simulink model "Generic_Aero_Piston_Digital_Twin"  (R2026a)
settings: Solver=VariableStepAuto  StopTime=30
libraries: SignalEditorBlockLib x3
settings Model: Creator=bhanu  LastModifiedBy=bhanu

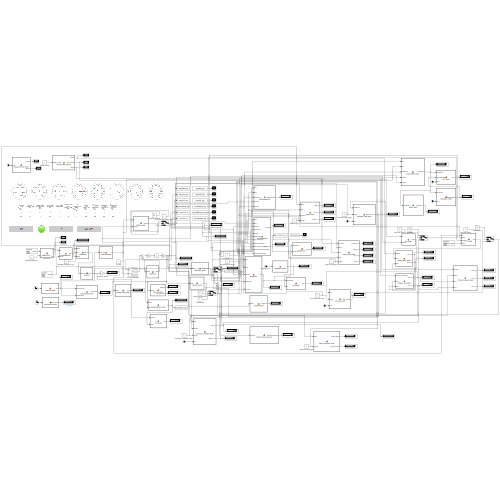
[thumbnail: Simulink's stored preview of the top-level diagram]
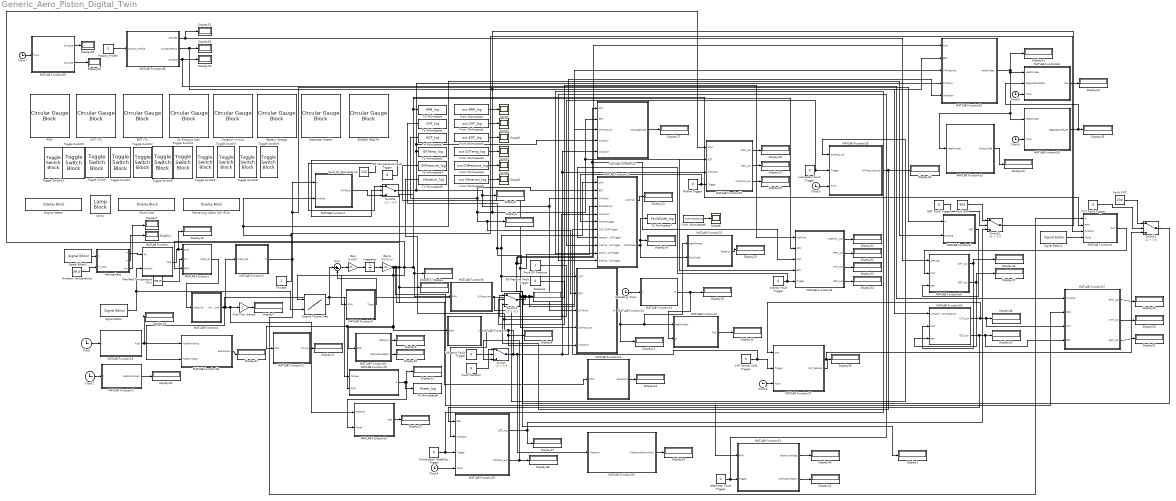
== system Generic_Aero_Piston_Digital_Twin ==
  " Fault Code" : DisplayBlock  LabelPosition=Hide  Transparency=1  GridColor=[0.502, 0.502, 0.502]
  Alternator Fault Trigger : Constant  Value=0
  Alternator Health : CircularGaugeBlock  LabelPosition=Hide  FontColor=[0.0, 0.0, 0.0]
  Ambient Temperature : Constant  Value=288.15
  Atmosphere : MATLAB Function  TreatAsAtomicUnit=on
  Battery Voltage : CircularGaugeBlock  LabelPosition=Hide  ScaleMax=16  FontColor=[0.0, 0.0, 0.0]
  CHT (°C) : CircularGaugeBlock  Description=CHT  LabelPosition=Hide  ScaleMax=150  FontColor=[0.0, 0.0, 0.0]
  CHT Fault Trigger : Constant  Value=0
  CHT Sensor Drift Trigger : Constant  Value=0
  Clock{,1..7} (8 alike) : Clock
  Combustion Instability Trigger : Constant  Value=0
  Display{,1..56} (57 alike) : Display
  EGT (°C) : CircularGaugeBlock  LabelPosition=Hide  ScaleMax=1000  FontColor=[0.0, 0.0, 0.0]
  EGT Fault Trigger : Constant  Value=0
  ENGINE HEALTH : CircularGaugeBlock  LabelPosition=Hide  FontColor=[0.0, 0.0, 0.0]
  "Engine Health  " : DisplayBlock  LabelPosition=Hide  Transparency=1  GridColor=[0.502, 0.502, 0.502]
  Engine Torque Map : Lookup_n-D  BreakpointsForDimension1=[3500 4000 4500 5000 5500 5800]  BreakpointsForDimension2=[0 0.25 0.5 0.75 1]  Table=|  InternalRulePriority=Speed  RndMeth=Simplest
      | [20 35 55 80 100;
      |  20 40 60 85 110;
      |  18 42 65 90 118;
      |  18 45 70 100 125;
      |  18 45 72 102 127.6;
      |  15 42 68 98 120]
      settings: InputPortMap=u0,u1
  Fault CHT : Constant  Value=130
  Fault EGT : Constant  Value=900
  Fault Oil Pressure : Constant
  Fault Oil Temperature : Constant  Value=120
  Fault Vibration : Constant  Value=5
  From Workspace : FromWorkspace  VariableName=out.RPM_log
  From Workspace1 : FromWorkspace  VariableName=out.CHT_log
  From Workspace2 : FromWorkspace  VariableName=out.EGT_log
  From Workspace3 : FromWorkspace  VariableName=out.OilTemp_log
  From Workspace4 : FromWorkspace  VariableName=out.OilPressure_log
  From Workspace5 : FromWorkspace  VariableName=out.Vibration_log
  From Workspace6 : FromWorkspace  VariableName=out.FaultCode_log
  Fuel Flow Sensor : Gain
  Gain : Gain  Gain=6.6667
  Gain1 : Gain  Gain=60/(2*pi)
  Injector Fault Trigger : Constant  Value=0
  Integrator : Integrator  InitialCondition=575.96
  Lamp : LampBlock  LabelPosition=Hide  DefaultColor=[192.0, 192.0, 192.0]
  Lubrication Fault Trigger : Constant  Value=0
  MATLAB Function : MATLAB Function  TreatAsAtomicUnit=on
  MATLAB Function1 : MATLAB Function  TreatAsAtomicUnit=on
  MATLAB Function10 : MATLAB Function  TreatAsAtomicUnit=on
  MATLAB Function11 : MATLAB Function  TreatAsAtomicUnit=on
  MATLAB Function12 : MATLAB Function  TreatAsAtomicUnit=on
  MATLAB Function13 : MATLAB Function  TreatAsAtomicUnit=on
  MATLAB Function14 : MATLAB Function  TreatAsAtomicUnit=on
  MATLAB Function15 : MATLAB Function  TreatAsAtomicUnit=on
  MATLAB Function16 : MATLAB Function  TreatAsAtomicUnit=on
  MATLAB Function17 : MATLAB Function  TreatAsAtomicUnit=on
  MATLAB Function18 : MATLAB Function  TreatAsAtomicUnit=on
  MATLAB Function19 : MATLAB Function  TreatAsAtomicUnit=on
  MATLAB Function2 : MATLAB Function  TreatAsAtomicUnit=on
  MATLAB Function20 : MATLAB Function  TreatAsAtomicUnit=on
  MATLAB Function21 : MATLAB Function  TreatAsAtomicUnit=on
  MATLAB Function22 : MATLAB Function  TreatAsAtomicUnit=on
  MATLAB Function23 : MATLAB Function  TreatAsAtomicUnit=on
  MATLAB Function24 : MATLAB Function  TreatAsAtomicUnit=on
  MATLAB Function25 : MATLAB Function  TreatAsAtomicUnit=on
  MATLAB Function26 : MATLAB Function  TreatAsAtomicUnit=on
  MATLAB Function27 : MATLAB Function  TreatAsAtomicUnit=on
  MATLAB Function28 : MATLAB Function  TreatAsAtomicUnit=on
  MATLAB Function29 : MATLAB Function  TreatAsAtomicUnit=on
  MATLAB Function3 : MATLAB Function  TreatAsAtomicUnit=on
  MATLAB Function30 : MATLAB Function  TreatAsAtomicUnit=on
  MATLAB Function31 : MATLAB Function  TreatAsAtomicUnit=on
  MATLAB Function32 : MATLAB Function  TreatAsAtomicUnit=on
  MATLAB Function33 : MATLAB Function  TreatAsAtomicUnit=on
  MATLAB Function34 : MATLAB Function  TreatAsAtomicUnit=on
  MATLAB Function35 : MATLAB Function  TreatAsAtomicUnit=on
  MATLAB Function36 : MATLAB Function  TreatAsAtomicUnit=on
  MATLAB Function37 : MATLAB Function  TreatAsAtomicUnit=on
  MATLAB Function38 : MATLAB Function  TreatAsAtomicUnit=on
  MATLAB Function39 : MATLAB Function  TreatAsAtomicUnit=on
  MATLAB Function4 : MATLAB Function  TreatAsAtomicUnit=on
  MATLAB Function5 : MATLAB Function  TreatAsAtomicUnit=on
  MATLAB Function6 : MATLAB Function  TreatAsAtomicUnit=on
  MATLAB Function7 : MATLAB Function  TreatAsAtomicUnit=on
  MATLAB Function8 : MATLAB Function  TreatAsAtomicUnit=on
  MATLAB Function9 : MATLAB Function  TreatAsAtomicUnit=on
  Manifold Temperature (Tm) : Constant  Value=288.15
  Misfire Trigger : Constant  Value=0
  Mission_Profile : Constant  Value=2
  Oil Pressure (bar) : CircularGaugeBlock  LabelPosition=Hide  ScaleMax=6  FontColor=[0.0, 0.0, 0.0]
  Oil Pressure Fault Trigger : Constant  Value=0
  Oil Temperature Fault Trigger : Constant  Value=0
  Operating Time : Clock
  RPM : CircularGaugeBlock  Tag=RPM  LabelPosition=Hide  ScaleMax=6000  FontColor=[0.0, 0.0, 0.0]
  Remaining Useful Life (RUL) : DisplayBlock  LabelPosition=Hide  Transparency=1  GridColor=[0.502, 0.502, 0.502]
  Scope{,1..6} (7 alike) : Scope
      Scope settings: ActiveDisplayYMinimum=3492.7664069639277  ActiveDisplayYMaximum=5723.0402452178787
      Scope1 settings: ActiveDisplayYMinimum=46.717948241029276  ActiveDisplayYMaximum=72.103645266326225
      Scope2 settings: ActiveDisplayYMinimum=420.76922361543927  ActiveDisplayYMaximum=801.55467899489327  DataLoggingVariableName=ScopeData2
      Scope3 settings: ActiveDisplayYMinimum=10  ActiveDisplayYMaximum=210  DataLoggingVariableName=ScopeData3
      Scope4 settings: ActiveDisplayYMinimum=3.4945760109784914  ActiveDisplayYMaximum=5.1672693321135013  DataLoggingVariableName=ScopeData4
      Scope5 settings: ActiveDisplayYMinimum=1.6286979532535071  ActiveDisplayYMaximum=2.0301472441392181  DataLoggingVariableName=ScopeData5
      Scope6 settings: ActiveDisplayYMinimum=-0.2207253886010363  ActiveDisplayYMaximum=0.19585492227979273  DataLoggingVariableName=ScopeData6
  Signal Editor : SignalEditorBlockLib/Signal Editor  FileName=C:\Users\bhanu\Documents\MATLAB\digital twin.mat  ActiveScenario=Scenario  ActiveSignal=Throttle  IsBus=off  OutputBusObjectStr=Bus: BusObject  SampleTime=0  ZeroCross=off  OutputAfterFinalValue=Setting to zero  Unit=inherit  PreserveSignalName=on  ApplySigPropsToAllScenarios=on  ApplySigPropsToAllSignals=off  SignalPropertySource=Dialog parameters
  Signal Editor1 : SignalEditorBlockLib/Signal Editor  FileName=C:\Users\bhanu\Documents\MATLAB\Amb Temp.mat  ActiveScenario=Scenario  ActiveSignal=Ambient Temp  IsBus=off  OutputBusObjectStr=Bus: BusObject  SampleTime=0  ZeroCross=off  OutputAfterFinalValue=Setting to zero  Unit=inherit  PreserveSignalName=on  ApplySigPropsToAllScenarios=on  ApplySigPropsToAllSignals=off  SignalPropertySource=Dialog parameters
  Signal Editor2 : SignalEditorBlockLib/Signal Editor  FileName=C:\Users\bhanu\Documents\MATLAB\Altitude.mat  ActiveScenario=Scenario  ActiveSignal=Altitude  IsBus=off  OutputBusObjectStr=Bus: BusObject  SampleTime=0  ZeroCross=off  OutputAfterFinalValue=Setting to zero  Unit=inherit  PreserveSignalName=on  ApplySigPropsToAllScenarios=on  ApplySigPropsToAllSignals=off  SignalPropertySource=Dialog parameters
  Sum : Sum  Inputs=|+-
  Switch{,1..4} (5 alike) : Switch  Criteria=u2 > Threshold  Threshold=0.5  SaturateOnIntegerOverflow=off  InputSameDT=off
  Throttle : Constant
  To Workspace : ToWorkspace  VariableName=RPM_log  SaveFormat=Timeseries  SampleTime=-1
  To Workspace1 : ToWorkspace  VariableName=CHT_log  SaveFormat=Timeseries  SampleTime=-1
  To Workspace2 : ToWorkspace  VariableName=EGT_log  SaveFormat=Timeseries  SampleTime=-1
  To Workspace3 : ToWorkspace  VariableName=OilTemp_log  SaveFormat=Timeseries  SampleTime=-1
  To Workspace4 : ToWorkspace  VariableName=OilPressure_log  SaveFormat=Timeseries  SampleTime=-1
  To Workspace5 : ToWorkspace  VariableName=Vibration_log  SaveFormat=Timeseries  SampleTime=-1
  To Workspace6 : ToWorkspace  VariableName=Power_log  SaveFormat=Timeseries  SampleTime=-1
  To Workspace7 : ToWorkspace  VariableName=FaultCode_log  SaveFormat=Timeseries  SampleTime=-1
  Toggle Switch{,1..10} (11 alike) : ToggleSwitchBlock
  Vibration (mm/s) : CircularGaugeBlock  LabelPosition=Hide  ScaleMax=5  FontColor=[0.0, 0.0, 0.0]
  Vibration Fault Trigger : Constant  Value=0
  wires:
  Ambient Temperature/1 -> Atmosphere/2(T_input)
  Atmosphere/1(P) -> MATLAB Function/1(Pa)
  Atmosphere/2(T) -> Display1/1
  Atmosphere/3(rho) -> Display2/1
  MATLAB Function/1(MAP) -> Display18/1, MATLAB Function1/1(MAP)
  Manifold Temperature (Tm)/1 -> MATLAB Function1/2(Tm)
  MATLAB Function1/1(mdot_air) -> MATLAB Function2/1(mdot_air)
  MATLAB Function2/1(mdot_fuel) -> MATLAB Function26/1(FuelFlow), MATLAB Function18/2(FuelBurnRate), MATLAB Function20/1(FuelFlow), Fuel Flow Sensor/1, MATLAB Function3/1(mdot_fuel)
  Engine Torque Map/1 -> Sum/1, MATLAB Function19/1(Torque)
  Sum/1 -> Gain/1
  Gain/1 -> Integrator/1
  Integrator/1 -> Gain1/1
  Gain1/1 -> MATLAB Function9/1(RPM), MATLAB Function10/1(RPM), MATLAB Function19/2(RPM), MATLAB Function11/1(RPM), MATLAB Function5/1(RPM), MATLAB Function37/2(RPM), MATLAB Function31/1(RPM), MATLAB Function25/1(RPM), Display17/1, MATLAB Function21/1(RPM), Engine Torque Map/1, MATLAB Function1/3(RPM), MATLAB Function4/2(RPM), To Workspace/1, MATLAB Function8/1(RPM), Display/1, MATLAB Function26/2(RPM)
  MATLAB Function5/1(Tload) -> Sum/2
  Throttle/1 -> MATLAB Function7/2(throttle), MATLAB Function6/2(throttle), MATLAB Function4/3(throttle)
  MATLAB Function3/1(P) -> MATLAB Function7/1(P), MATLAB Function6/1(P), MATLAB Function4/1(P)
  Switch1/1 -> MATLAB Function32/1(CHT), MATLAB Function23/1(CHT), MATLAB Function26/3(CHT), To Workspace1/1, MATLAB Function12/1(CHT), Display3/1, MATLAB Function13/1(CHT)
  Switch2/1 -> MATLAB Function12/2(EGT), Display4/1, MATLAB Function13/2(EGT), To Workspace2/1, MATLAB Function23/2(EGT), MATLAB Function25/2(EGT), MATLAB Function26/4(EGT), MATLAB Function32/2(EGT)
  Switch4/1 -> MATLAB Function32/4(OilTemp), MATLAB Function23/4(OilTemp), To Workspace3/1, MATLAB Function12/3(OilTemp), MATLAB Function13/3(OilTemp), Display5/1
  Switch3/1 -> To Workspace4/1, MATLAB Function13/4(OilPressure), MATLAB Function12/4(OilPressure), MATLAB Function23/3(OilPressure), MATLAB Function32/3(OilPressure), Display6/1
  Fuel Flow Sensor/1 -> Display7/1
  Switch/1 -> MATLAB Function32/5(Vibration), MATLAB Function25/3(Vibration), MATLAB Function23/5(Vibration), MATLAB Function30/1(Vibration), To Workspace5/1, MATLAB Function13/5(Vibration), MATLAB Function12/5(Vibration), Display8/1
  MATLAB Function10/1(BatteryV) -> Display9/1
  MATLAB Function10/2(AlternatorHealth) -> Display10/1
  MATLAB Function11/1(timing) -> Display11/1
  MATLAB Function12/1(HI) -> MATLAB Function22/1(HealthIndex), MATLAB Function14/1(HealthIndex), Display12/1
  MATLAB Function13/1(Anomaly) -> Display13/1
  MATLAB Function13/2(FaultCode) -> To Workspace7/1, Display14/1, MATLAB Function22/2(FaultCode)
  MATLAB Function14/1(RUL) -> Display15/1
  Operating Time/1 -> MATLAB Function15/1(t)
  MATLAB Function15/1(D) -> MATLAB Function14/2(D), Display16/1
  Signal Editor/1 -> Engine Torque Map/2, MATLAB Function/2(throttle)
  From Workspace/1 -> Scope/1
  From Workspace1/1 -> Scope1/1
  From Workspace2/1 -> Scope2/1
  From Workspace3/1 -> Scope3/1
  From Workspace4/1 -> Scope4/1
  From Workspace5/1 -> Scope5/1
  Signal Editor1/1 -> MATLAB Function4/4(Tamb)
  Signal Editor2/1 -> Atmosphere/1(h)
  Clock/1 -> MATLAB Function16/1(t)
  MATLAB Function16/1(Fuel) -> Display19/1, MATLAB Function18/1(FuelRemaining)
  Clock1/1 -> MATLAB Function17/1(t)
  MATLAB Function17/1(FuelConsumed) -> Display20/1
  MATLAB Function18/1(Endurance) -> Display21/1
  MATLAB Function19/1(P) -> MATLAB Function20/2(Power), Display22/1, To Workspace6/1
  MATLAB Function20/1(SFC) -> Display23/1
  MATLAB Function21/1(Response) -> Display24/1
  MATLAB Function22/1(Severity) -> Display25/1
  From Workspace6/1 -> Scope6/1
  Vibration Fault Trigger/1 -> Switch/2
  Fault Vibration/1 -> Switch/1
  Fault CHT/1 -> Switch1/1
  CHT Fault Trigger/1 -> Switch1/2
  Fault EGT/1 -> Switch2/1
  EGT Fault Trigger/1 -> Switch2/2
  Fault Oil Pressure/1 -> Switch3/1
  Oil Pressure Fault Trigger/1 -> Switch3/2
  MATLAB Function7/1(OilTemp) -> Switch4/3
  Fault Oil Temperature/1 -> Switch4/1
  Oil Temperature Fault Trigger/1 -> Switch4/2
  MATLAB Function23/1(MessageCode) -> Display27/1
  Misfire Trigger/1 -> MATLAB Function13/6(MisfireTrigger), MATLAB Function25/4(Trigger)
  MATLAB Function25/1(RPM_out) -> Display28/1
  MATLAB Function25/3(Vibration_out) -> Display30/1
  MATLAB Function25/2(EGT_out) -> Display29/1
  Injector Fault Trigger/1 -> MATLAB Function13/8(InjectorFaultTrigger), MATLAB Function26/5(Trigger)
  MATLAB Function26/1(FuelFlow_out) -> Display31/1
  MATLAB Function26/4(EGT_out) -> Display34/1
  MATLAB Function26/3(CHT_out) -> Display33/1
  MATLAB Function26/2(RPM_out) -> Display32/1
  CHT Sensor Drift Trigger/1 -> MATLAB Function13/7(CHT_DriftTrigger), MATLAB Function27/2(Trigger)
  Clock2/1 -> MATLAB Function27/3(Time)
  MATLAB Function27/1(CHT_Sensed) -> Switch1/3, Display35/1
  Lubrication Fault Trigger/1 -> MATLAB Function13/9(LubricationFaultTrigger), MATLAB Function28/2(Trigger)
  Clock3/1 -> MATLAB Function28/3(Time)
  MATLAB Function8/1(OilPressure) -> MATLAB Function28/1(OilPressure)
  MATLAB Function28/1(OilPressure_out) -> Display36/1, Switch3/3
  Combustion Instability Trigger/1 -> MATLAB Function13/10(CombustionInstabilityTrigger), MATLAB Function29/3(Trigger)
  MATLAB Function29/1(EGT_out) -> Display37/1, Switch2/3
  Clock4/1 -> MATLAB Function29/4(Time)
  MATLAB Function9/1(V) -> MATLAB Function29/2(Vibration)
  MATLAB Function29/2(Vibration_out) -> Switch/3, Display38/1
  MATLAB Function30/1(VibrationPatternFault) -> Display39/1
  Alternator Fault Trigger/1 -> MATLAB Function13/11(AlternatorFaultTrigger), MATLAB Function31/2(Trigger)
  MATLAB Function31/2(AlternatorHealth) -> Display41/1
  MATLAB Function31/1(BatteryVoltage) -> Display40/1
  MATLAB Function32/1(HealthIndex) -> MATLAB Function35/1(HealthIndex), MATLAB Function33/1(HealthIndex), MATLAB Function34/1(HealthIndex), Display42/1
  MATLAB Function33/1(StatusCode) -> Display43/1
  MATLAB Function34/1(RUL) -> Display44/1
  Clock5/1 -> MATLAB Function35/2(Time)
  MATLAB Function35/1(DegradationRate) -> MATLAB Function34/2(DegradationRate), Display45/1
  Clock6/1 -> MATLAB Function34/3(Time)
  MATLAB Function36/1(CHT_out) -> MATLAB Function24/2(CHT), Display46/1
  MATLAB Function36/2(EGT_out) -> MATLAB Function24/3(EGT), Display47/1
  MATLAB Function4/1(CHT) -> MATLAB Function36/2(CHT)
  MATLAB Function6/1(EGT) -> MATLAB Function36/3(EGT)
  MATLAB Function24/1(CHT_out) -> MATLAB Function27/1(CHT), MATLAB Function37/3(CHT), Display48/1
  MATLAB Function24/2(EGT_out) -> MATLAB Function29/1(EGT), MATLAB Function37/4(EGT), Display26/1
  MATLAB Function37/1(RPM_out) -> Display49/1
  MATLAB Function37/2(CHT_out) -> Display50/1
  MATLAB Function37/3(EGT_out) -> Display51/1
  Mission_Profile/1 -> MATLAB Function38/1(Mission_Profile)
  MATLAB Function38/2(AmbientTemp) -> Display53/1, MATLAB Function24/1(Ambient_Temperature)
  MATLAB Function38/3(Throttle) -> MATLAB Function37/1(Throttle), Display54/1
  MATLAB Function38/1(Altitude) -> Display52/1, MATLAB Function36/1(Altitude)
  Clock7/1 -> MATLAB Function39/1(Time)
  MATLAB Function39/1(Throttle) -> Display55/1
  MATLAB Function39/2(Altitude) -> Display56/1

== matlab function Generic_Aero_Piston_Digital_Twin/MATLAB Function10 ==
  data: RPM input; BatteryV output; AlternatorHealth output
function [BatteryV, AlternatorHealth] = Electrical_Model(RPM)

BatteryV = 24;

if RPM >= 1500
    AlternatorHealth = 100;
else
    AlternatorHealth = 50;
end

== matlab function Generic_Aero_Piston_Digital_Twin/MATLAB Function11 ==
  data: RPM input; timing output
function timing = InjectionTiming_Model(RPM)

timing_base = 25;      % degrees BTDC
timing = timing_base + 0.001*(RPM - 5500);

== matlab function Generic_Aero_Piston_Digital_Twin/MATLAB Function12 ==
  data: CHT input; HI output; EGT input; OilTemp input; OilPressure input; Vibration input
function HI = HealthIndex(CHT, EGT, OilTemp, OilPressure, Vibration)

HI = 100;

if CHT > 120
    HI = HI - 15;
end

if EGT > 850
    HI = HI - 15;
end

if OilTemp > 110
    HI = HI - 10;
end

if OilPressure < 2
    HI = HI - 20;
end

if Vibration > 4
    HI = HI - 20;
end

HI = max(0,HI);

== matlab function Generic_Aero_Piston_Digital_Twin/MATLAB Function13 ==
  data: CHT input; Anomaly output; EGT input; OilTemp input; OilPressure input; Vibration input; FaultCode output; MisfireTrigger input; CHT_DriftTrigger input; InjectorFaultTrigger input; LubricationFaultTrigger input; CombustionInstabilityTrigger input; AlternatorFaultTrigger input
function [Anomaly,FaultCode] = AnomalyDetection(CHT,EGT,OilTemp,OilPressure,Vibration,MisfireTrigger,CHT_DriftTrigger,InjectorFaultTrigger,LubricationFaultTrigger,CombustionInstabilityTrigger,AlternatorFaultTrigger)

Anomaly = 0;
FaultCode = 0;

% Misfire
if MisfireTrigger > 0.5
    Anomaly = 1;
    FaultCode = 6;

% CHT Sensor Drift
elseif CHT_DriftTrigger > 0.5
    Anomaly = 1;
    FaultCode = 7;

% Injector Abnormality
elseif InjectorFaultTrigger > 0.5
    Anomaly = 1;
    FaultCode = 8;

% Lubrication Degradation
elseif LubricationFaultTrigger > 0.5
    Anomaly = 1;
    FaultCode = 9;

% Combustion Instability
elseif CombustionInstabilityTrigger > 0.5
    Anomaly = 1;
    FaultCode = 10;

% Battery / Alternator Fault
elseif AlternatorFaultTrigger > 0.5
    Anomaly = 1;
    FaultCode = 11;

% High CHT
elseif CHT > 120
    Anomaly = 1;
    FaultCode = 1;

% High EGT
elseif EGT > 850
    Anomaly = 1;
    FaultCode = 2;

% Low Oil Pressure
elseif OilPressure < 2
    Anomaly = 1;
    FaultCode = 3;

% High Oil Temperature
elseif OilTemp > 110
    Anomaly = 1;
    FaultCode = 4;

% High Vibration
elseif Vibration > 4
    Anomaly = 1;
    FaultCode = 5;
end

== matlab function Generic_Aero_Piston_Digital_Twin/MATLAB Function14 ==
  data: HealthIndex input; RUL output; D input
function RUL = RUL_Model(HealthIndex,D)

InitialLife = 1000;   % hours

RUL = InitialLife * (HealthIndex/100) * (1-D);

RUL = max(0,RUL);

== matlab function Generic_Aero_Piston_Digital_Twin/MATLAB Function15 ==
  data: t input; D output
function D = Degradation_Model(t)

t_hours = t/3600;

degradation_rate = 0.00005;

D = degradation_rate * t_hours;

D = min(D,1);

== matlab function Generic_Aero_Piston_Digital_Twin/MATLAB Function16 ==
  data: t input; Fuel output
function Fuel = FuelLevel_Model(t)

Fuel_initial = 25;      % kg
Fuel_burn_rate = 0.004821;  % kg/s

Fuel = Fuel_initial - Fuel_burn_rate*t;
Fuel = max(0,Fuel);

== matlab function Generic_Aero_Piston_Digital_Twin/MATLAB Function17 ==
  data: t input; FuelConsumed output
function FuelConsumed = FuelConsumed_Model(t)

FuelBurnRate = 0.004821;   % kg/s

FuelConsumed = FuelBurnRate*t;

== matlab function Generic_Aero_Piston_Digital_Twin/MATLAB Function18 ==
  data: FuelRemaining input; Endurance output; FuelBurnRate input
function Endurance = FuelEndurance_Model(FuelRemaining, FuelBurnRate)

if FuelBurnRate > 0
    Endurance = FuelRemaining / FuelBurnRate;
else
    Endurance = 0;
end

== matlab function Generic_Aero_Piston_Digital_Twin/MATLAB Function ==
  data: Pa input; MAP output; throttle input
function MAP = ManifoldPressure(Pa, throttle)

MAP = Pa * (1 + 0.35 * throttle);

== matlab function Generic_Aero_Piston_Digital_Twin/MATLAB Function19 ==
  data: Torque input; P output; RPM input
function P = MechanicalPower_Model(Torque,RPM)

omega = 2*pi*RPM/60;

P = Torque*omega;

== matlab function Generic_Aero_Piston_Digital_Twin/MATLAB Function20 ==
  data: FuelFlow input; SFC output; Power input
function SFC = SFC_Model(FuelFlow,Power)

if Power > 0
    Power_kW = Power/1000;
    SFC = (FuelFlow*3600)/Power_kW;
else
    SFC = 0;
end

== matlab function Generic_Aero_Piston_Digital_Twin/MATLAB Function21 ==
  data: RPM input; Response output
function Response = ThrottleResponse(RPM)

RPM_initial = 5500;

Response = abs(RPM - RPM_initial);

== matlab function Generic_Aero_Piston_Digital_Twin/MATLAB Function22 ==
  data: HealthIndex input; Severity output; FaultCode input
function Severity = FaultSeverity(HealthIndex,FaultCode)

Severity = 0;

if FaultCode ~= 0
    if HealthIndex < 50
        Severity = 2;       % Critical
    else
        Severity = 1;       % Warning
    end
end

== matlab function Generic_Aero_Piston_Digital_Twin/MATLAB Function23 ==
  data: CHT input; MessageCode output; EGT input; OilPressure input; OilTemp input; Vibration input
function MessageCode = FaultMessageCode(CHT,EGT,OilPressure,OilTemp,Vibration)

MessageCode = 0;

if CHT > 120
    MessageCode = 1;
end

if EGT > 850
    MessageCode = 2;
end

if OilPressure < 2
    MessageCode = 3;
end

if OilTemp > 110
    MessageCode = 4;
end

if Vibration > 4
    MessageCode = 5;
end

== matlab function Generic_Aero_Piston_Digital_Twin/MATLAB Function24 ==
  data: Ambient_Temperature input; CHT_out output; CHT input; EGT input; EGT_out output
function [CHT_out,EGT_out] = Ambient_Temp_Effect(Ambient_Temperature,CHT,EGT)

CHT_out = CHT;
EGT_out = EGT;

if Ambient_Temperature > 40
    CHT_out = CHT + 5;
    EGT_out = EGT + 8;
elseif Ambient_Temperature > 30
    CHT_out = CHT + 2;
    EGT_out = EGT + 4;
end

== matlab function Generic_Aero_Piston_Digital_Twin/MATLAB Function25 ==
  data: RPM input; RPM_out output; EGT input; Vibration input; Trigger input; EGT_out output; Vibration_out output
function [RPM_out,EGT_out,Vibration_out] = Misfire_Model(RPM,EGT,Vibration,Trigger)

RPM_out = RPM;
EGT_out = EGT;
Vibration_out = Vibration;

if Trigger > 0.5
    RPM_out = RPM * 0.90;
    EGT_out = EGT * 0.92;
    Vibration_out = Vibration + 2.5;
end

== matlab function Generic_Aero_Piston_Digital_Twin/MATLAB Function26 ==
  data: FuelFlow input; FuelFlow_out output; RPM input; CHT input; EGT input; Trigger input; RPM_out output; CHT_out output; EGT_out output
function [FuelFlow_out,RPM_out,CHT_out,EGT_out] = Injector_Fault_Model(FuelFlow,RPM,CHT,EGT,Trigger)

FuelFlow_out = FuelFlow;
RPM_out = RPM;
CHT_out = CHT;
EGT_out = EGT;

if Trigger > 0.5
    FuelFlow_out = FuelFlow * 1.15;
    RPM_out = RPM * 0.95;
    CHT_out = CHT + 8;
    EGT_out = EGT + 30;
end

== matlab function Generic_Aero_Piston_Digital_Twin/Atmosphere ==
  data: h input; P output; T_input input; T output; rho output
function [P,T,rho] = Atmosphere(h,T_input)

T0 = 288.15;       % Sea-level temperature (K)
P0 = 101325;       % Sea-level pressure (Pa)
L  = 0.0065;       % Temperature lapse rate (K/m)
g  = 9.80665;      % Gravity (m/s^2)
R  = 287.05;       % Air gas constant (J/kg/K)

% Standard atmosphere temperature
T_std = T0 - L*h;

% Use supplied ambient temperature if provided
if h == 0
    T = T_input;
else
    T = T_std;
end

% Pressure
P = P0*(T/T0)^(g/(R*L));

% Density
rho = P/(R*T);

== matlab function Generic_Aero_Piston_Digital_Twin/MATLAB Function27 ==
  data: CHT input; CHT_Sensed output; Trigger input; Time input
function CHT_Sensed = CHT_Sensor_Drift(CHT,Trigger,Time)

CHT_Sensed = CHT;

if Trigger > 0.5
    CHT_Sensed = CHT + 0.2*Time;
end

== matlab function Generic_Aero_Piston_Digital_Twin/MATLAB Function28 ==
  data: OilPressure input; OilPressure_out output; Trigger input; Time input
function OilPressure_out = Lubrication_Fault_Model(OilPressure,Trigger,Time)

OilPressure_out = OilPressure;

if Trigger > 0.5
    OilPressure_out = OilPressure - 0.02*Time;
end

== matlab function Generic_Aero_Piston_Digital_Twin/MATLAB Function29 ==
  data: EGT input; EGT_out output; Vibration input; Trigger input; Time input; Vibration_out output
function [EGT_out,Vibration_out] = Combustion_Instability_Model(EGT,Vibration,Trigger,Time)

EGT_out = EGT;
Vibration_out = Vibration;

if Trigger > 0.5
    EGT_out = EGT + 20*sin(2*pi*0.5*Time);
    Vibration_out = Vibration + 1.5;
end

== matlab function Generic_Aero_Piston_Digital_Twin/MATLAB Function30 ==
  data: Vibration input; VibrationPatternFault output
function VibrationPatternFault = Vibration_Pattern_Detector(Vibration)

VibrationPatternFault = 0;

if Vibration > 3.5
    VibrationPatternFault = 1;
end

== matlab function Generic_Aero_Piston_Digital_Twin/MATLAB Function31 ==
  data: RPM input; BatteryVoltage output; Trigger input; AlternatorHealth output
function [BatteryVoltage,AlternatorHealth] = Battery_Alternator_Model(RPM,Trigger)

BatteryVoltage = 14.0;
AlternatorHealth = 100;

if RPM < 2500
    BatteryVoltage = 12.5;
    AlternatorHealth = 70;
end

if Trigger > 0.5
    BatteryVoltage = 11.5;
    AlternatorHealth = 40;
end

== matlab function Generic_Aero_Piston_Digital_Twin/MATLAB Function32 ==
  data: CHT input; HealthIndex output; EGT input; OilPressure input; OilTemp input; Vibration input
function HealthIndex = Engine_Health_Index(CHT,EGT,OilPressure,OilTemp,Vibration)

HealthIndex = 100;

% CHT penalty
if CHT > 100
    HealthIndex = HealthIndex - (CHT - 100) * 0.3;
end

% EGT penalty
if EGT > 700
    HealthIndex = HealthIndex - (EGT - 700) * 0.03;
end

% Oil pressure penalty
if OilPressure < 3
    HealthIndex = HealthIndex - (3 - OilPressure) * 10;
end

% Oil temperature penalty
if OilTemp > 90
    HealthIndex = HealthIndex - (OilTemp - 90) * 0.2;
end

% Vibration penalty
if Vibration > 2
    HealthIndex = HealthIndex - (Vibration - 2) * 5;
end

% Limit health index
if HealthIndex > 100
    HealthIndex = 100;
elseif HealthIndex < 0
    HealthIndex = 0;
end

== matlab function Generic_Aero_Piston_Digital_Twin/MATLAB Function33 ==
  data: HealthIndex input; StatusCode output
function StatusCode = Health_Status(HealthIndex)

if HealthIndex >= 90
    StatusCode = 1;       % HEALTHY

elseif HealthIndex >= 70
    StatusCode = 2;       % WARNING

elseif HealthIndex >= 50
    StatusCode = 3;       % DEGRADED

else
    StatusCode = 4;       % CRITICAL
end

== matlab function Generic_Aero_Piston_Digital_Twin/MATLAB Function34 ==
  data: HealthIndex input; RUL output; DegradationRate input; Time input
function RUL = RUL_Model(HealthIndex,DegradationRate,Time)

MaxLife = 2000;

HealthBasedRUL = MaxLife * (HealthIndex / 100);

TimePenalty = DegradationRate * Time;

RUL = HealthBasedRUL - TimePenalty;

if RUL < 0
    RUL = 0;
elseif RUL > MaxLife
    RUL = MaxLife;
end

== matlab function Generic_Aero_Piston_Digital_Twin/MATLAB Function35 ==
  data: HealthIndex input; DegradationRate output; Time input
function DegradationRate = Degradation_Model(HealthIndex,Time)

BaseRate = 0.01;

if HealthIndex >= 90
    DegradationRate = BaseRate;
elseif HealthIndex >= 70
    DegradationRate = BaseRate * 2;
elseif HealthIndex >= 50
    DegradationRate = BaseRate * 4;
else
    DegradationRate = BaseRate * 6;
end

== matlab function Generic_Aero_Piston_Digital_Twin/MATLAB Function36 ==
  data: Altitude input; CHT_out output; CHT input; EGT input; EGT_out output
function [CHT_out,EGT_out] = Altitude_Effect_Model(Altitude,CHT,EGT)

CHT_out = CHT;
EGT_out = EGT;

if Altitude > 5000
    CHT_out = CHT + 5;
    EGT_out = EGT + 10;
elseif Altitude > 2000
    CHT_out = CHT + 2;
    EGT_out = EGT + 5;
end

== matlab function Generic_Aero_Piston_Digital_Twin/MATLAB Function37 ==
  data: Throttle input; RPM_out output; RPM input; CHT input; EGT input; CHT_out output; EGT_out output
function [RPM_out,CHT_out,EGT_out] = Throttle_Transition_Model(Throttle,RPM,CHT,EGT)

RPM_out = RPM;
CHT_out = CHT;
EGT_out = EGT;

if Throttle > 80
    RPM_out = RPM + 500;
    CHT_out = CHT + 5;
    EGT_out = EGT + 15;

elseif Throttle < 30
    RPM_out = RPM - 300;
    CHT_out = CHT - 2;
    EGT_out = EGT - 5;
end

== matlab function Generic_Aero_Piston_Digital_Twin/MATLAB Function1 ==
  data: MAP input; mdot_air output; Tm input; RPM input
function mdot_air = AirMassFlow(MAP, Tm, RPM)

Vd = 0.0011;       % Engine displacement, m^3
eta_v = 0.85;      % Volumetric efficiency
R = 287.05;        % Air gas constant

omega = RPM / 60;

mdot_air = eta_v * MAP * Vd * omega / (2 * R * Tm);

== matlab function Generic_Aero_Piston_Digital_Twin/MATLAB Function38 ==
  data: Mission_Profile input; Altitude output; AmbientTemp output; Throttle output
function [Altitude,AmbientTemp,Throttle] = Mission_Profile_Selector(Mission_Profile)

% Default values
Altitude = 0;
AmbientTemp = 25;
Throttle = 50;

if Mission_Profile == 1
    % Normal Cruise
    Altitude = 1000;
    AmbientTemp = 25;
    Throttle = 50;

elseif Mission_Profile == 2
    % High Altitude
    Altitude = 6000;
    AmbientTemp = 15;
    Throttle = 60;

elseif Mission_Profile == 3
    % Hot Weather
    Altitude = 1000;
    AmbientTemp = 45;
    Throttle = 60;

elseif Mission_Profile == 4
    % Rapid Throttle
    Altitude = 1000;
    AmbientTemp = 25;
    Throttle = 90;

elseif Mission_Profile == 5
    % Endurance
    Altitude = 5000;
    AmbientTemp = 20;
    Throttle = 55;
end

== matlab function Generic_Aero_Piston_Digital_Twin/MATLAB Function39 ==
  data: Time input; Throttle output; Altitude output
function [Throttle,Altitude] = Endurance_Profile_Model(Time)

if Time < 60
    % Climb
    Throttle = 70;
    Altitude = 2000;

elseif Time < 120
    % Cruise
    Throttle = 55;
    Altitude = 5000;

elseif Time < 180
    % Endurance cruise
    Throttle = 50;
    Altitude = 5000;

else
    % Descent
    Throttle = 40;
    Altitude = 2000;
end

== matlab function Generic_Aero_Piston_Digital_Twin/MATLAB Function2 ==
  data: mdot_air input; mdot_fuel output
function mdot_fuel = FuelFlow(mdot_air)

AFR = 14.7;

mdot_fuel = mdot_air / AFR;

== matlab function Generic_Aero_Piston_Digital_Twin/MATLAB Function3 ==
  data: mdot_fuel input; P output
function P = CombustionPower(mdot_fuel)

LHV = 43e6;       % Fuel lower heating value, J/kg
eta_b = 0.30;     % Brake thermal efficiency

P = mdot_fuel * LHV * eta_b;

== matlab function Generic_Aero_Piston_Digital_Twin/MATLAB Function4 ==
  data: P input; CHT output; RPM input; throttle input; Tamb input
function CHT = CHT_Model(P, RPM, throttle, Tamb)

CHT_ambient = Tamb - 273.15;
K = 0.0008;

CHT = CHT_ambient + K * P * throttle;

== matlab function Generic_Aero_Piston_Digital_Twin/MATLAB Function5 ==
  data: RPM input; Tload output
function Tload = LoadTorque(RPM)

Tload_rated = 127.6;
RPM_rated = 5500;

Tload = Tload_rated * (RPM/RPM_rated)^2;

== matlab function Generic_Aero_Piston_Digital_Twin/MATLAB Function6 ==
  data: P input; EGT output; throttle input
function EGT = EGT_Model(P, throttle)

EGT_ambient = 20;
K = 0.012;

EGT = EGT_ambient + K * P * throttle;

== matlab function Generic_Aero_Piston_Digital_Twin/MATLAB Function7 ==
  data: P input; OilTemp output; throttle input
function OilTemp = OilTemp_Model(P, throttle)

OilTemp_ambient = 20;
OilTemp_max = 110;

OilTemp = OilTemp_ambient + ...
    (OilTemp_max - OilTemp_ambient) * throttle;

== matlab function Generic_Aero_Piston_Digital_Twin/MATLAB Function8 ==
  data: RPM input; OilPressure output
function OilPressure = OilPressure_Model(RPM)

P_idle = 2;        % bar
P_rated = 5;       % bar
RPM_idle = 1500;
RPM_rated = 5500;

OilPressure = P_idle + ...
    (P_rated - P_idle) * ...
    (RPM - RPM_idle)/(RPM_rated - RPM_idle);

OilPressure = max(P_idle, min(P_rated, OilPressure));

== matlab function Generic_Aero_Piston_Digital_Twin/MATLAB Function9 ==
  data: RPM input; V output
function V = Vibration_Model(RPM)

V_base = 1.0;
K = 0.00018;

V = V_base + K * RPM;
